simulink model "fulladderdesign"  (R2014a)
settings: Solver=ode45  StartTime=0.0  StopTime=10.0  RelTol=1e-3
settings Model: Creator=Andrew  LastModifiedBy=Andrew

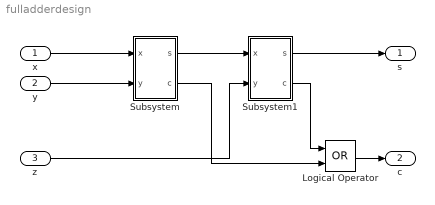
== system fulladderdesign ==
  x : Inport
  y : Inport  Port=2
  z : Inport  Port=3
  Logical Operator : Logic  Operator=OR  AllPortsSameDT=off  OutDataTypeStr=boolean
  Subsystem : Subsystem
  Subsystem1 : Subsystem
  s : Outport
  c : Outport  Port=2
  wires:
  x/1 -> Subsystem/1(x)
  y/1 -> Subsystem/2(y)
  Logical Operator/1 -> c/1
  Subsystem1/2(c) -> Logical Operator/1
  Subsystem/2(c) -> Logical Operator/2
  z/1 -> Subsystem1/2(y)
  Subsystem/1(s) -> Subsystem1/1(x)
  Subsystem1/1(s) -> s/1

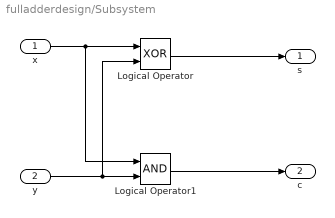
== system fulladderdesign/Subsystem ==
  x : Inport
  y : Inport  Port=2
  Logical Operator : Logic  Operator=XOR  AllPortsSameDT=off  OutDataTypeStr=boolean
  Logical Operator1 : Logic  AllPortsSameDT=off  OutDataTypeStr=boolean
  s : Outport
  c : Outport  Port=2
  wires:
  x/1 -> Logical Operator1/1, Logical Operator/1
  Logical Operator1/1 -> c/1
  y/1 -> Logical Operator/2, Logical Operator1/2
  Logical Operator/1 -> s/1

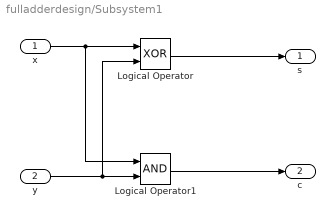
== system fulladderdesign/Subsystem1 ==
  x : Inport
  y : Inport  Port=2
  Logical Operator : Logic  Operator=XOR  AllPortsSameDT=off  OutDataTypeStr=boolean
  Logical Operator1 : Logic  AllPortsSameDT=off  OutDataTypeStr=boolean
  s : Outport
  c : Outport  Port=2
  wires:
  x/1 -> Logical Operator1/1, Logical Operator/1
  Logical Operator1/1 -> c/1
  y/1 -> Logical Operator/2, Logical Operator1/2
  Logical Operator/1 -> s/1
